simulink model "rigid_body_fdyn_HC_LuGre"  (Simulink 8.5)
settings: Solver=ode4  StartTime=0.0  StopTime=10.0  FixedStep=1.000000e-04  MaxStep=1e-4  MinStep=1e-6  RelTol=1e-4  AbsTol=1e-4
values from neighbouring files (symbols this model uses):
  HC_params = [R,h,alpha]'    [HuntCrossley_LuGre_1DOF_example.m]
  LuGre_kv_arctan = 10    [HuntCrossley_LuGre_1DOF_example.m]
  LuGre_params = [1000, 100, 0.1, 0.8, 0.9, 20, 1]'    [HuntCrossley_LuGre_1DOF_example.m]
  r_B_C_ges = allcomb([l1/2;-l1/2], [l2/2;-l2/2], [l3/2;-l3/2])'    [HuntCrossley_LuGre_1DOF_example.m]
  Ts = 1e-4    (= 0.0001)    [HuntCrossley_LuGre_1DOF_example.m]
libraries: lib_rigidbody_dynamics_mapletb_mod x2
settings Model: Creator=schappler  LastModifiedBy=schappler
settings DataIOCC: LimitDataPoints=off  SaveFormat=StructureWithTime  SignalLoggingSaveFormat=Dataset
settings OptimizationCC: ExpressionDepthLimit=128
settings DebuggingCC: UnderspecifiedInitializationDetection=Simplified  MergeDetectMultiDrivingBlocksExec=error  FcnCallInpInsideContextMsg=EnableAllAsError  StateNameClashWarn=none
settings GRTTargetCC: CombineOutputUpdateFcns=on  GRTInterface=off

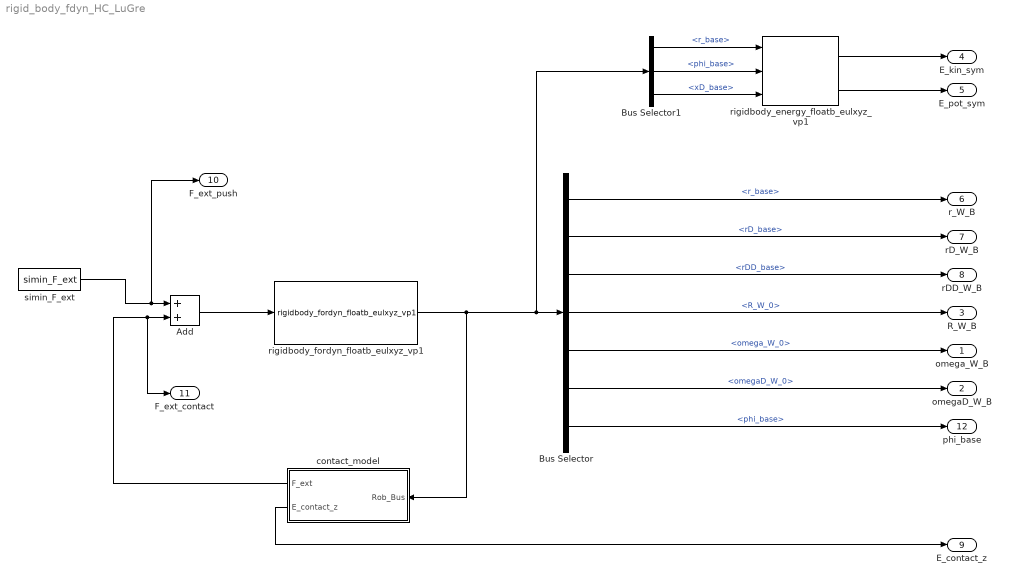
== system rigid_body_fdyn_HC_LuGre ==
  Add : Sum
  Bus Selector : BusSelector  OutputSignals=r_base,rD_base,rDD_base,R_W_0,omega_W_0,omegaD_W_0,phi_base
  Bus Selector1 : BusSelector  OutputSignals=r_base,phi_base,xD_base
  contact_model : Subsystem  Variant=on
  rigidbody_energy_floatb_eulxyz_vp1 : lib_rigidbody_dynamics_mapletb_mod/rigidbody_energy_floatb_eulxyz_vp1  KinPar_mdh=KinPar_mdh  DynPar1=DynPar1  g_world=g_W
  rigidbody_fordyn_floatb_eulxyz_vp1 : lib_rigidbody_dynamics_mapletb_mod/rigidbody_fordyn_floatb_eulxyz_vp1  r_base_t0=r_t0  rD_base_t0=rD_t0  phi_base_t0=phi_base_t0  phiD_base_t0=phiD_base_t0  g_world=g_W  KinPar_mdh=KinPar_mdh  DynPar1=DynPar1
  simin_F_ext : FromWorkspace  VariableName=simin_F_ext  SampleTime=0  Interpolate=off  OutputAfterFinalValue=Holding final value
  omega_W_B : Outport
  omegaD_W_B : Outport  Port=2
  R_W_B : Outport  Port=3
  E_kin_sym : Outport  Port=4
  E_pot_sym : Outport  Port=5
  r_W_B : Outport  Port=6
  rD_W_B : Outport  Port=7
  rDD_W_B : Outport  Port=8
  E_contact_z : Outport  Port=9
  F_ext_push : Outport  Port=10  PortDimensions=6
  F_ext_contact : Outport  Port=11  PortDimensions=6
  phi_base : Outport  Port=12
  wires:
  rigidbody_fordyn_floatb_eulxyz_vp1/1 -> contact_model/1(Rob_Bus), Bus Selector1/1, Bus Selector/1
  Bus Selector/1 -> r_W_B/1  "<r_base>"
  Bus Selector/3 -> rDD_W_B/1  "<rDD_base>"
  Bus Selector/5 -> omega_W_B/1  "<omega_W_0>"
  Bus Selector/6 -> omegaD_W_B/1  "<omegaD_W_0>"
  Bus Selector/2 -> rD_W_B/1  "<rD_base>"
  Bus Selector/4 -> R_W_B/1  "<R_W_0>"
  rigidbody_energy_floatb_eulxyz_vp1/1 -> E_kin_sym/1
  rigidbody_energy_floatb_eulxyz_vp1/2 -> E_pot_sym/1
  Bus Selector1/3 -> rigidbody_energy_floatb_eulxyz_vp1/3  "<xD_base>"
  Bus Selector1/1 -> rigidbody_energy_floatb_eulxyz_vp1/1  "<r_base>"
  Bus Selector1/2 -> rigidbody_energy_floatb_eulxyz_vp1/2  "<phi_base>"
  simin_F_ext/1 -> F_ext_push/1, Add/1
  Add/1 -> rigidbody_fordyn_floatb_eulxyz_vp1/1
  contact_model/1(F_ext) -> F_ext_contact/1, Add/2
  contact_model/2(E_contact_z) -> E_contact_z/1
  Bus Selector/7 -> phi_base/1  "<phi_base>"

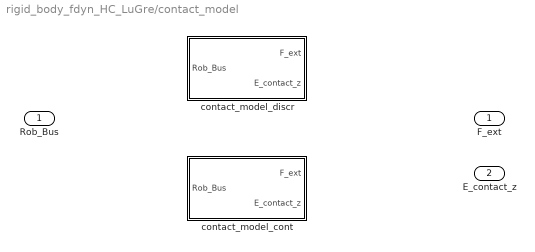
== system rigid_body_fdyn_HC_LuGre/contact_model ==
  Rob_Bus : Inport
  contact_model_cont : Subsystem  VariantControl=CONTACT_CONTI
  contact_model_discr : Subsystem  VariantControl=CONTACT_DISCR
  F_ext : Outport  PortDimensions=6
  E_contact_z : Outport  Port=2  PortDimensions=1

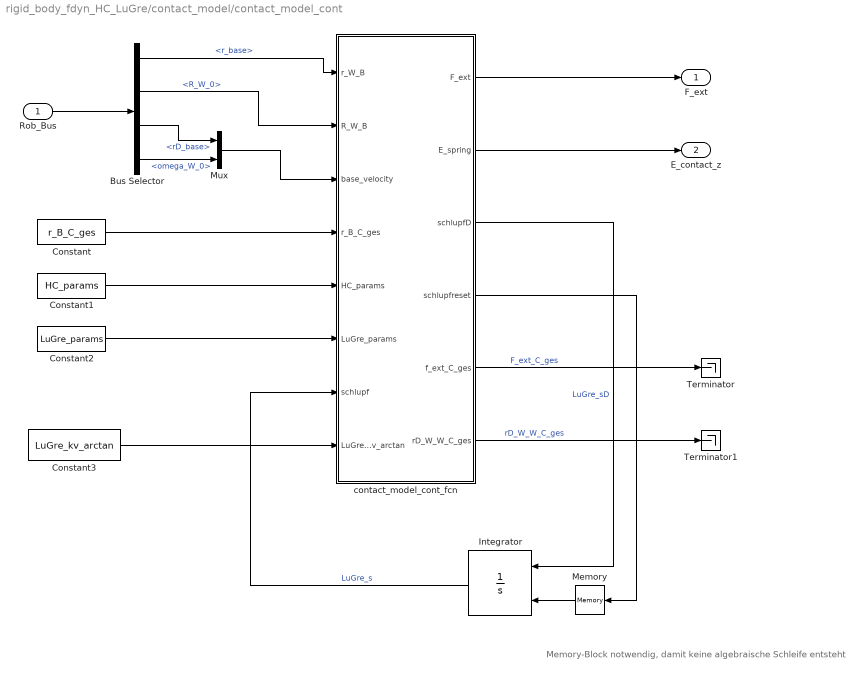
== system rigid_body_fdyn_HC_LuGre/contact_model/contact_model_cont ==
  note: Memory-Block notwendig, damit keine algebraische Schleife entsteht
  Rob_Bus : Inport
  Bus Selector : BusSelector  OutputSignals=r_base,R_W_0,rD_base,omega_W_0
  Constant : Constant  Value=r_B_C_ges
  Constant1 : Constant  Value=HC_params
  Constant2 : Constant  Value=LuGre_params
  Constant3 : Constant  Value=LuGre_kv_arctan
  Integrator : Integrator  ExternalReset=rising
  Memory : Memory
  Mux : Mux  Inputs=2
  Terminator : Terminator
  Terminator1 : Terminator
  contact_model_cont_fcn : MATLAB Function  SystemSampleTime=Ts
  F_ext : Outport  PortDimensions=6
  E_contact_z : Outport  Port=2  PortDimensions=1
  wires:
  Rob_Bus/1 -> Bus Selector/1
  Bus Selector/3 -> Mux/1  "<rD_base>"
  Bus Selector/4 -> Mux/2  "<omega_W_0>"
  Constant/1 -> contact_model_cont_fcn/4(r_B_C_ges)
  Constant1/1 -> contact_model_cont_fcn/5(HC_params)
  Constant2/1 -> contact_model_cont_fcn/6(LuGre_params)
  Bus Selector/2 -> contact_model_cont_fcn/2(R_W_B)  "<R_W_0>"
  Mux/1 -> contact_model_cont_fcn/3(base_velocity)
  contact_model_cont_fcn/1(F_ext) -> F_ext/1
  contact_model_cont_fcn/2(E_spring) -> E_contact_z/1
  Bus Selector/1 -> contact_model_cont_fcn/1(r_W_B)  "<r_base>"
  Integrator/1 -> contact_model_cont_fcn/7(schlupf)  "LuGre_s"
  contact_model_cont_fcn/3(schlupfD) -> Integrator/1  "LuGre_sD"
  contact_model_cont_fcn/5(f_ext_C_ges) -> Terminator/1  "F_ext_C_ges"
  contact_model_cont_fcn/6(rD_W_W_C_ges) -> Terminator1/1  "rD_W_W_C_ges"
  Constant3/1 -> contact_model_cont_fcn/8(LuGre_kv_arctan)
  contact_model_cont_fcn/4(schlupfreset) -> Memory/1
  Memory/1 -> Integrator/2

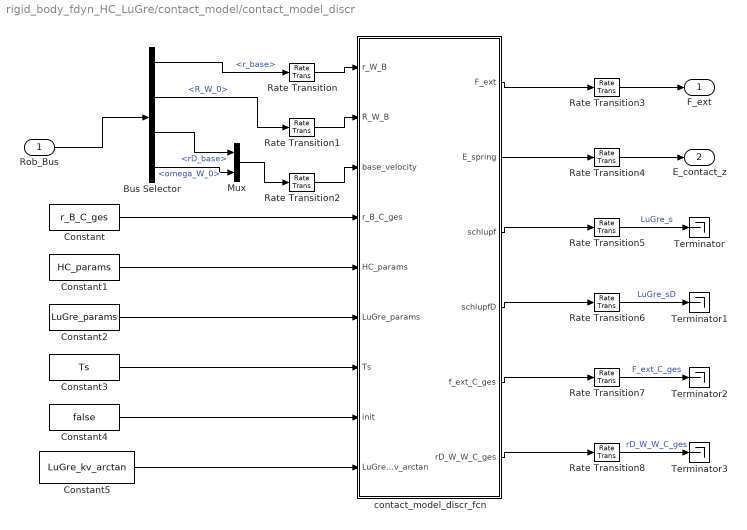
== system rigid_body_fdyn_HC_LuGre/contact_model/contact_model_discr ==
  Rob_Bus : Inport
  Bus Selector : BusSelector  OutputSignals=r_base,R_W_0,rD_base,omega_W_0
  Constant : Constant  Value=r_B_C_ges
  Constant1 : Constant  Value=HC_params
  Constant2 : Constant  Value=LuGre_params
  Constant3 : Constant  Value=Ts
  Constant4 : Constant  Value=false
  Constant5 : Constant  Value=LuGre_kv_arctan
  Mux : Mux  Inputs=2
  Rate Transition : RateTransition  OutPortSampleTime=Ts
  Rate Transition1 : RateTransition  OutPortSampleTime=Ts
  Rate Transition2 : RateTransition  OutPortSampleTime=Ts
  Rate Transition{3..8} (6 alike) : RateTransition  OutPortSampleTime=0
  Terminator{,1..3} (4 alike) : Terminator
  contact_model_discr_fcn : MATLAB Function  TreatAsAtomicUnit=on  SystemSampleTime=Ts
  F_ext : Outport  PortDimensions=6
  E_contact_z : Outport  Port=2  PortDimensions=1
  wires:
  Rob_Bus/1 -> Bus Selector/1
  Bus Selector/1 -> Rate Transition/1  "<r_base>"
  Bus Selector/2 -> Rate Transition1/1  "<R_W_0>"
  Mux/1 -> Rate Transition2/1
  Bus Selector/3 -> Mux/1  "<rD_base>"
  Bus Selector/4 -> Mux/2  "<omega_W_0>"
  Constant/1 -> contact_model_discr_fcn/4(r_B_C_ges)
  Constant1/1 -> contact_model_discr_fcn/5(HC_params)
  contact_model_discr_fcn/1(F_ext) -> Rate Transition3/1
  Constant2/1 -> contact_model_discr_fcn/6(LuGre_params)
  Constant3/1 -> contact_model_discr_fcn/7(Ts)
  Constant4/1 -> contact_model_discr_fcn/8(init)
  Rate Transition/1 -> contact_model_discr_fcn/1(r_W_B)
  Rate Transition1/1 -> contact_model_discr_fcn/2(R_W_B)
  Rate Transition2/1 -> contact_model_discr_fcn/3(base_velocity)
  Rate Transition3/1 -> F_ext/1
  contact_model_discr_fcn/2(E_spring) -> Rate Transition4/1
  Rate Transition4/1 -> E_contact_z/1
  contact_model_discr_fcn/3(schlupf) -> Rate Transition5/1
  contact_model_discr_fcn/4(schlupfD) -> Rate Transition6/1
  contact_model_discr_fcn/5(f_ext_C_ges) -> Rate Transition7/1
  contact_model_discr_fcn/6(rD_W_W_C_ges) -> Rate Transition8/1
  Constant5/1 -> contact_model_discr_fcn/9(LuGre_kv_arctan)
  Rate Transition5/1 -> Terminator/1  "LuGre_s"
  Rate Transition6/1 -> Terminator1/1  "LuGre_sD"
  Rate Transition7/1 -> Terminator2/1  "F_ext_C_ges"
  Rate Transition8/1 -> Terminator3/1  "rD_W_W_C_ges"

== matlab function contact_model/contact_model_cont/contact_model_cont_fcn ==
  data: F_ext output double; r_W_B input double; R_W_B input double; base_velocity input double; r_B_C_ges input double; HC_params input double; LuGre_params input double; schlupf input double; E_spring output double; schlupfD output double; schlupfreset output double; f_ext_C_ges output double; rD_W_W_C_ges output double; LuGre_kv_arctan input double
% Kontaktmodell mit Hunt-Crossley und Lugre
% Zeitdiskrete Implementierung
% 
% Siehe atlas5_foot_ground_force_Hunt_Crossley_LuGre.m

% Moritz Schappler, schappler@irt.uni-hannover.de, 2016-11
% (c) Institut für Regelungstechnik, Universität Hannover

function [F_ext, E_spring, schlupfD, schlupfreset, f_ext_C_ges, rD_W_W_C_ges] = fcn(r_W_B, R_W_B, base_velocity, ...
  r_B_C_ges, HC_params, LuGre_params, schlupf, LuGre_kv_arctan)
%#codegen

% Jeweils zwei aufeinanderfolgende Einträge für den Schlupf (xy) eines
% Punktes
schlupfD = zeros(2*200,1);
schlupfreset = false(2*200,1);

rD_W_W_B = base_velocity(1:3);
omega_W_B = base_velocity(4:6);
F_ext = zeros(6,1);
f_ext_C_ges = zeros(3,200);
rD_W_W_C_ges = zeros(3,200);
E_spring = 0;
% Gehe alle Kontaktpunkte durch
nC = size(r_B_C_ges,2);
for iC = 1:nC
  % Berechne Kinematik des Kontaktpunktes
  r_W_B_C = R_W_B * r_B_C_ges(:,iC);
  r_W_W_C = r_W_B + r_W_B_C;
  rD_W_W_C = rD_W_W_B + cross(omega_W_B, r_W_B_C);
  
  % Prüfe Kontakt
  d = -r_W_W_C(3);
  if d <= 0
    % Kein Kontakt
    schlupfreset((iC*2)-1:iC*2) = true; % Zurücksetzen Schlupf-Modell
    continue
  end
  
  % Berechne Kontaktmodell
  [F_s_norm,F_d_z, E_spring] = Hunt_Crossley_contact_model_func(d, -rD_W_W_C(3), ...
    HC_params(1), HC_params(2), HC_params(3));
  
  % Kontaktmodell Tangentialkraft
  [F_d_xy, sD_i] = LuGre_tangential_friction_model_func(rD_W_W_C(1:2), F_s_norm, ...
    schlupf((iC*2)-1:iC*2), LuGre_params, LuGre_kv_arctan);
  schlupfD((iC*2)-1:iC*2) = sD_i;
  
  F_d = [F_d_xy; F_d_z];
  F_s = F_s_norm * [0;0;1]; % Kraft per Definition senkrecht auf Ebene

  % Kontaktkraft (Steifigkeit und Dämpfung)
  VZ_Kraft = 1;
  F_contact = VZ_Kraft * (F_s+F_d);

  F_eff_W = [F_s+F_d; cross(r_W_B_C, F_contact)];

  F_ext = F_ext + F_eff_W;
  f_ext_C_ges(:,iC) = F_contact;   
  
  rD_W_W_C_ges(:,iC) = rD_W_W_C;
end

== matlab function contact_model/contact_model_discr/contact_model_discr_fcn ==
  data: F_ext output double; r_W_B input double; R_W_B input double; base_velocity input double; r_B_C_ges input double; HC_params input double; LuGre_params input double; Ts input double; init input double; E_spring output double; schlupf output double; schlupfD output double; f_ext_C_ges output double; rD_W_W_C_ges output double; LuGre_kv_arctan input double
% Kontaktmodell mit Hunt-Crossley und Lugre
% Zeitdiskrete Implementierung
% 
% Siehe atlas5_foot_ground_force_Hunt_Crossley_LuGre.m

% Moritz Schappler, schappler@irt.uni-hannover.de, 2016-11
% (c) Institut für Regelungstechnik, Universität Hannover

function [F_ext, E_spring, schlupf, schlupfD, f_ext_C_ges, rD_W_W_C_ges] = ...
  fcn(r_W_B, R_W_B, base_velocity, r_B_C_ges, HC_params, LuGre_params, Ts, init, LuGre_kv_arctan)
%#codegen

persistent schlupf_alt;
if isempty(schlupf_alt) || init
  schlupf_alt = zeros(2*200,1);
end
schlupf = zeros(2*200,1);
schlupfD = zeros(2*200,1);

rD_W_W_B = base_velocity(1:3);
omega_W_B = base_velocity(4:6);
F_ext = zeros(6,1);
f_ext_C_ges = zeros(3,200);
rD_W_W_C_ges = zeros(3,200);
E_spring = 0;
% Gehe alle Kontaktpunkte durch
nC = size(r_B_C_ges,2);
for iC = 1:nC
  % Berechne Kinematik des Kontaktpunktes
  r_W_B_C = R_W_B * r_B_C_ges(:,iC);
  r_W_W_C = r_W_B + r_W_B_C;
  rD_W_W_C = rD_W_W_B + cross(omega_W_B, r_W_B_C);
  
  % Prüfe Kontakt
  d = -r_W_W_C(3);
  if d <= 0
    % Kein Kontakt
    schlupf_alt((iC*2)-1:iC*2) = 0; % Zurücksetzen Schlupf-Modell
    schlupf((iC*2)-1:iC*2) = 0;
    continue
  end
  
  
  % Schlupf-Zustand bestimmen
  s_alt_i = schlupf_alt((iC*2)-1:iC*2);
  
  % Berechne Kontaktmodell
  [F_s_norm,F_d_z, E_spring] = Hunt_Crossley_contact_model_func(d, -rD_W_W_C(3), ...
    HC_params(1), HC_params(2), HC_params(3));
    
  % Kontaktmodell Tangentialkraft
  [F_d_xy, sD_i] = LuGre_tangential_friction_model_func(rD_W_W_C(1:2), F_s_norm, s_alt_i(1:2), LuGre_params, LuGre_kv_arctan);

  if any(abs(F_d_xy) > 2.7)
    1;
  end
  
  F_d = [F_d_xy; F_d_z];
  F_s = F_s_norm * [0;0;1]; % Kraft per Definition senkrecht auf Ebene

  % Kontaktkraft (Steifigkeit und Dämpfung)
  VZ_Kraft = 1;
  F_contact = VZ_Kraft * (F_s+F_d);

  F_eff_W = [F_s+F_d; cross(r_W_B_C, F_contact)];

  F_ext = F_ext + F_eff_W;
  f_ext_C_ges(:,iC) = F_contact;
  
  rD_W_W_C_ges(:,iC) = rD_W_W_C;
  
  % Schlupf aus Tangentialkraftmodell aufintegrieren
  s_neu_i = s_alt_i + Ts*sD_i;
  schlupf((iC*2)-1:iC*2) = s_neu_i;
  schlupfD((iC*2)-1:iC*2) = sD_i;
    
  
end

schlupf_alt = schlupf;
